simulink model "PDcontroller"  (R2019a)
settings: Solver=VariableStepAuto  StartTime=0.0  StopTime=20  RelTol=1e-3
undefined symbols (not defined in the file or in its folder): b, J, km
settings Model: Creator=user  LastModifiedBy=user

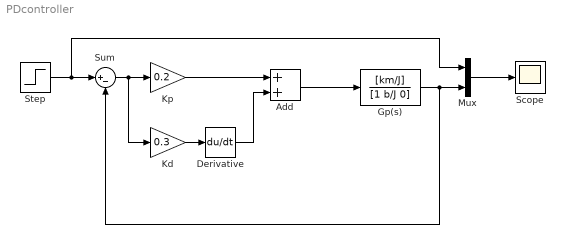
== system PDcontroller ==
  Add : Sum
  Derivative : Derivative
  Gp(s) : TransferFcn  Numerator=[km/J]  Denominator=[1 b/J 0]
  Kd : Gain  Gain=0.3
  Kp : Gain  Gain=0.2
  Mux : Mux  Inputs=2
  Scope : Scope
  Step : Step  After=2  SampleTime=0.1
  Sum : Sum  Inputs=|+-
  wires:
  Gp(s)/1 -> Mux/2, Sum/2
  Mux/1 -> Scope/1
  Step/1 -> Mux/1, Sum/1
  Sum/1 -> Kd/1, Kp/1
  Add/1 -> Gp(s)/1
  Kp/1 -> Add/1
  Kd/1 -> Derivative/1
  Derivative/1 -> Add/2
